simulink model "power_3phseriescomp"  (R2022a)
settings: Solver=FixedStepDiscrete  StartTime=0.0  StopTime=0.2  FixedStep=Ts  RelTol=1e-4  EnableMultiTasking=on
PreLoadFcn:
  | Ts=50e-6;
InitFcn:
  | Ts=50e-6;
undefined symbols (not defined in the file): D1, Delta, DiscIntNeverNeededParam
libraries: spsSeriesRLCBranchLib x6, spsBreakerLib x6, spsCurrentMeasurementLib x6, spsSurgeArresterLib x6, spsParallelRLCBranchLib x6, spsVoltageMeasurementLib x6, spsThreePhaseSeriesRLCLoadLib x4, spsLoadFlowBusLib x4, spsThreePhaseVIMeasurementLib x3, spsThreePhaseBreakerLib x2, spsDistributedParametersLineLib x2, spsThreePhaseSourceLib x1
(part 1 of 2)
settings Model: ExtModeTrigMode=oneshot  ExtModeArmWhenConnect=off  Creator=The MathWorks, Inc.  LastModifiedBy=thoma
settings SolverCC: AlgebraicLoopSolver=TrustRegion
settings DataIOCC: SaveFormat=Array  ReturnWorkspaceOutputs=off  SignalLoggingName=sigsOut
settings OptimizationCC: BlockReduction=off  BooleanDataType=off  ExpressionDepthLimit=2147483647  InitFltsAndDblsToZero=on  EfficientMapNaN2IntZero=off  LifeSpan=inf
settings DebuggingCC: UnderspecifiedInitializationDetection=Classic  MergeDetectMultiDrivingBlocksExec=none  CheckExecutionContextPreStartOutputMsg=on  SignalResolutionControl=TryResolveAllWithWarning  MultiTaskDSMMsg=warning  MultiTaskCondExecSysMsg=none  FcnCallInpInsideContextMsg=warning  UnconnectedLineMsg=warning  StateNameClashWarn=warning  SFUnexpectedBacktrackingDiag=warning  SFNoUnconditionalDefaultTransitionDiag=warning  SFExecutionAtInitializationDiag=none  SFMachineParentedDataDiag=warning  ArithmeticOperatorsInVariantConditions=warning
settings HardwareCC: ProdBitPerPointer=32  ProdBitPerSizeT=32  ProdBitPerPtrDiffT=32  ProdLargestAtomicFloat=None  ProdIntDivRoundTo=Undefined  ProdEndianess=Unspecified  ProdWordSize=32  ProdHWDeviceType=Specified  TargetUnknown=on
settings ModelReferenceCC: PropagateSignalLabelsOutOfModel=off
settings SFSimCC: SimUseLocalCustomCode=off  CustomCodeUndefinedFunction=UseInterfaceOnly
settings RTWCC: RTWUseLocalCustomCode=off  DLArmComputeVersion=19.05
settings CodeAppCC: StateflowObjectComments=on
settings GRTTargetCC: TargetLangStandard=C89/C90 (ANSI)  CombineOutputUpdateFcns=off  GRTInterface=on
settings ConfigComp: CovMetricSettings=dw  CovSaveCumulativeToWorkspaceVar=on  CovSaveSingleToWorkspaceVar=on  CovExternalEMLEnable=off  CovSFcnEnable=off
settings SimscapeCC: SimscapeNormalizeSystem=off

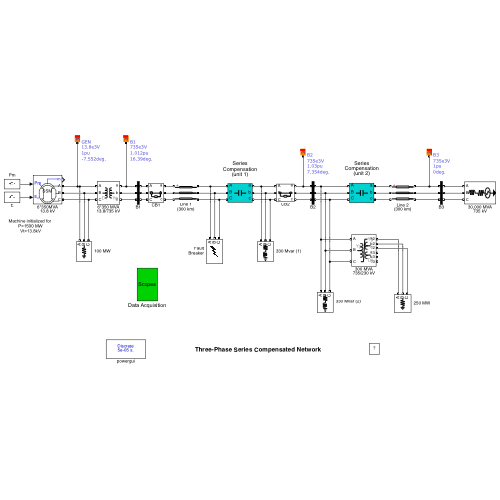
[thumbnail: Simulink's stored preview of the top-level diagram]
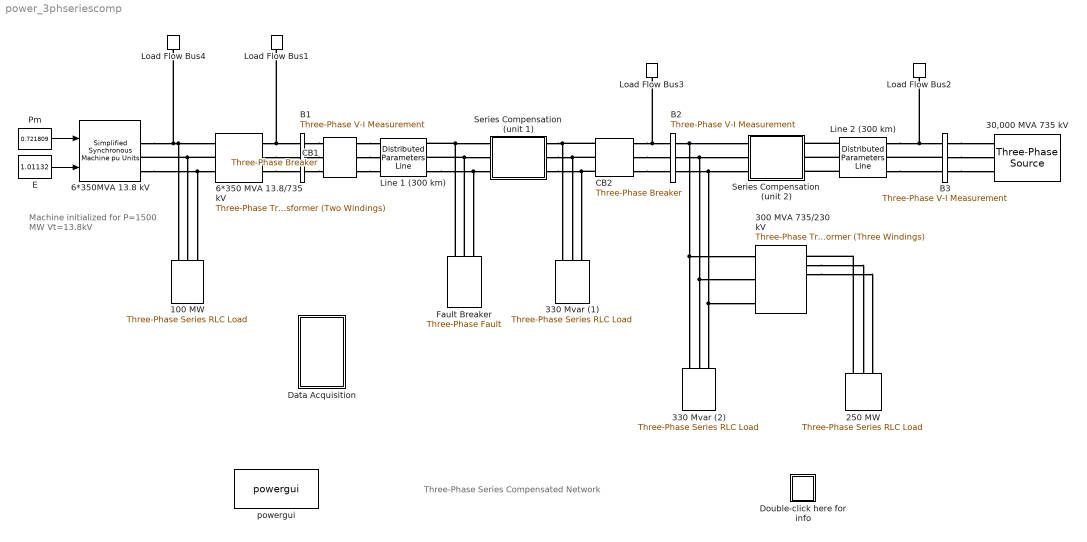
== system power_3phseriescomp ==
  note: Machine initialized for
      |  P=1500 MW
      |  Vt=13.8kV
  note: Three-Phase Series Compensated Network
  100 MW : spsThreePhaseSeriesRLCLoadLib/Three-Phase Series RLC Load  LConnTagsString=A|B|C  Configuration=Y (grounded)  NominalVoltage=13.8e3  Vabc=[1e3 1e3 1e3]  Vabcp=[1e3 1e3 1e3]  NominalFrequency=60  UnbalancedPower=off  ActivePower=100000000  InductivePower=0  CapacitivePower=0  Pabc=[10e3 9e3 11e3]  QLabc=[100 90 110]  QCabc=[100 90 110]  Pabcp=[10e3 9e3 11e3]  QLabcp=[100 90 110]  QCabcp=[100 90 110]  Measurements=None  LoadType=constant Z
  250 MW : spsThreePhaseSeriesRLCLoadLib/Three-Phase Series RLC Load  LConnTagsString=A|B|C  Configuration=Y (grounded)  NominalVoltage=230e3  Vabc=[1e3 1e3 1e3]  Vabcp=[1e3 1e3 1e3]  NominalFrequency=60  UnbalancedPower=off  ActivePower=250000000  InductivePower=0  CapacitivePower=0  Pabc=[10e3 9e3 11e3]  QLabc=[100 90 110]  QCabc=[100 90 110]  Pabcp=[10e3 9e3 11e3]  QLabcp=[100 90 110]  QCabcp=[100 90 110]  Measurements=None  LoadType=constant Z
  30,000 MVA 735 kV : spsThreePhaseSourceLib/Three-Phase Source  InternalConnection=Yg  VoltagePhases=off  Voltage=(735000)*0.98865  PhaseAngle=-2.0892  Voltage_phases=[25e3 25e3 25e3]/sqrt(3)  PhaseAngles_phases=[0 -120 +120]  Frequency=60  NonIdealSource=on  SpecifyImpedance=on  Resistance=735^2/30000/10  Inductance=735^2/30000/377  ShortCircuitLevel=30000e6  BaseVoltage=735e3  XRratio=10  BusType=swing  Pref=0  Qref=0  Prefabc=[10e3, 10e3, 10e3]  Qrefabc=[0, 0, 0]  Qmin=-Inf  Qmax=Inf
  300 MVA 735/230 kV : spsThreePhaseTransformerThreeWindingsLib/Three-Phase Transformer (Three Windings)  Winding1Connection=Yg  Winding2Connection=Yg  Winding3Connection=Delta (D1)  CoreType=Three single-phase transformers  SetSaturation=on  Hysteresis=off  DataFile='hysteresis'  SetInitialFlux=off  Measurements=None  UNITS=pu  NominalPower=[ 300e6 , 60 ]  Winding1=[ 735e3 , 0.002 , 0.15 ]  Winding2=[ 230e3 , 0.002 , 0 ]  Winding3=[ 25e3 , 0.05 , 0.20 ]  Rm=500  Lm=1000  L0=0.5  Saturation="[  0,0  ;  0.0012,1.2  ;  1.0,1.45 ]"  InitialFluxes=[-1.02015948080927 0.506449133666726 0.513710347142541]  BreakLoop=on  DiscreteSolver=Trapezoidal iterative  DataType=off  TransfoNumber=0
      settings: AttributesFormatString=\n  SourceProductBaseCode=PS
  330 Mvar (1) : spsThreePhaseSeriesRLCLoadLib/Three-Phase Series RLC Load  LConnTagsString=A|B|C  Configuration=Y (grounded)  NominalVoltage=735e3  Vabc=[1e3 1e3 1e3]  Vabcp=[1e3 1e3 1e3]  NominalFrequency=60  UnbalancedPower=off  ActivePower=1320000  InductivePower=330e6  CapacitivePower=0  Pabc=[10e3 9e3 11e3]  QLabc=[100 90 110]  QCabc=[100 90 110]  Pabcp=[10e3 9e3 11e3]  QLabcp=[100 90 110]  QCabcp=[100 90 110]  Measurements=None  LoadType=constant Z
  "330 Mvar (2) " : spsThreePhaseSeriesRLCLoadLib/Three-Phase Series RLC Load  LConnTagsString=A|B|C  Configuration=Y (grounded)  NominalVoltage=735e3  Vabc=[1e3 1e3 1e3]  Vabcp=[1e3 1e3 1e3]  NominalFrequency=60  UnbalancedPower=off  ActivePower=1320000  InductivePower=330e6  CapacitivePower=0  Pabc=[10e3 9e3 11e3]  QLabc=[100 90 110]  QCabc=[100 90 110]  Pabcp=[10e3 9e3 11e3]  QLabcp=[100 90 110]  QCabcp=[100 90 110]  Measurements=None  LoadType=constant Z
  6*350 MVA 13.8/735 kV : spsThreePhaseTransformerTwoWindingsLib/Three-Phase Transformer (Two Windings)  Winding1Connection=Delta (D1)  Winding2Connection=Yg  CoreType=Three single-phase transformers  SetSaturation=off  Hysteresis=off  DataFile='hysteresis'  SetInitialFlux=off  Measurements=None  UNITS=pu  NominalPower=[ 6*350e6 , 60 ]  Winding1=[ 13.8e3 , 0.002 , 0.08 ]  Winding2=[ 735e3 , 0.002 , 0.08 ]  Rm=500  Lm=500  L0=0.5  Saturation=[ 0,0 ; 0.0024,1.2 ; 1.0,1.52 ]  InitialFluxes=[ 0.8 , -0.8 , 0.7 ]  BreakLoop=off  DiscreteSolver=Trapezoidal iterative  DataType=off  TransfoNumber=0
  6*350MVA 13.8 kV : spsSimplifiedSynchronousMachinepuUnitsLib/Simplified Synchronous Machine pu Units  ConnectionType=3-wire Y  MechanicalLoad=Mechanical power Pm  MeasurementBus=off  NominalParameters="[ 6*350e6 13.8e3  60 ]"  Mechanical=[ inf,0,2 ]  InternalRL="[ 0.22/15  0.22 ]"  InitialConditions=[0 1.43122 0.716215 0.716215 0.716215 -3.34575 -123.346 116.654 ]  IterativeDiscreteModel=Trapezoidal non iterative  TsBlock=-1  TsPowergui=0  LoadFlowParameters=[1,0,0,0,0]  Units=0  BusType=PV  Pref=1500000000  Qref=0  Qmin=-Inf  Qmax=Inf  PLF=0  QLF=0
      settings: AttributesFormatString=\n  SourceProductBaseCode=PS
  B1 : spsThreePhaseVIMeasurementLib/Three-Phase V-I Measurement  VoltageMeasurement=phase-to-ground  SetLabelV=on  LabelV=Vabc_B1  Vpu=on  VpuLL=off  CurrentMeasurement=yes  SetLabelI=on  LabelI=Iabc_B1  Ipu=on  Pbase=100e6  Vbase=735e3  OutputType=Complex  PhasorSimulation=off  PSBequivalent=0
  B2 : spsThreePhaseVIMeasurementLib/Three-Phase V-I Measurement  VoltageMeasurement=phase-to-ground  SetLabelV=on  LabelV=Vabc_B2  Vpu=on  VpuLL=off  CurrentMeasurement=yes  SetLabelI=on  LabelI=Iabc_B2  Ipu=on  Pbase=100e6  Vbase=735e3  OutputType=Complex  PhasorSimulation=off  PSBequivalent=0
  B3 : spsThreePhaseVIMeasurementLib/Three-Phase V-I Measurement  VoltageMeasurement=no  SetLabelV=on  LabelV=Vabc_B3  Vpu=on  VpuLL=off  CurrentMeasurement=no  SetLabelI=on  LabelI=Iabc_B3  Ipu=on  Pbase=100e6  Vbase=735e3  OutputType=Complex  PhasorSimulation=off  PSBequivalent=0
  CB1 : spsThreePhaseBreakerLib/Three-Phase Breaker  InitialState=closed  SwitchA=on  SwitchB=on  SwitchC=on  SwitchTimes="[5/60  ]"  External=off  BreakerResistance=0.001  SnubberResistance=1e5  SnubberCapacitance=inf  Measurements=None
      settings: AttributesFormatString=\n
  CB2 : spsThreePhaseBreakerLib/Three-Phase Breaker  InitialState=closed  SwitchA=on  SwitchB=on  SwitchC=on  SwitchTimes="[5/60  ]"  External=off  BreakerResistance=0.001  SnubberResistance=1e5  SnubberCapacitance=inf  Measurements=None
      settings: AttributesFormatString=\n
  Data Acquisition : Subsystem  mask(Data Acquisition){}
      mask Display: disp('Scopes')
  Double-click here for info : Subsystem
      settings: OpenFcn=showdemo(bdroot(gcb))
      mask Display: disp('?')
  E : Constant  Value=1.01132
  Fault Breaker : spsThreePhaseFaultLib/Three-Phase Fault  InitialStates=0  FaultA=on  FaultB=off  FaultC=off  GroundFault=on  SwitchTimes=[ 1/60 6/60]  External=off  SwitchStatus=NaN  FaultResistance=0.001  GroundResistance=1  SnubberResistance=inf  SnubberCapacitance=inf  Measurements=Fault currents
  Line 1 (300 km) : spsDistributedParametersLineLib/Distributed Parameters Line  Phases=3  Length=300  Frequency=60  Resistance=[0.01273 0.3864]  Inductance="[0.9337e-3  4.1264e-3]"  Capacitance=[12.74e-9 7.751e-9]  x1=[-0.0017 -9.8128912515287e-08 0 0;-0.00165 -9.90072730950498e-08 0 0;-0.0016 -9.98504568621167e-08 0 0;-0.00155 -1.0065816423731e-07 0 0;-0.0015 -1.01430108246046e-07 0 0;-0.00145 -1.02166014620294e-07 0 0;-0.0014 -1.02865621896022e-07 0 0;-0.00135 -1.03528681506097e-07 0 0;-0.0013 -1.04154957868598e-07 0 0;-0.00125 -1.04744228470514e-07 0 0;-0.0012 -1.05296283946806e-07 0 0;-0.00115 -1.05810928154793e-07 0 0;-0.0011 -1.06287978243837e-07 0 0;-0.00105 -1.06727264720314e-07 298982.565692147 -680729.342896261;-0.001 -1.07128631507831e-07 311760.155284911 -674973.083751637;-0.00095 -1.07491936002678e-07 324426.977978985 -668977.009884319;-0.0009 -1.07817049124499e-07 336978.53331258 -662743.251670802;-0.00085 -1.0810385536215e-07 349410.361777853 -656274.023935697;-0.0008 -1.0835225281474e-07 361718.046405344 -649571.625164814;-0.00075 -1.08562153227837e-07 373897.214333311 -642638.436688521;-0.0007 -1.08733482024824e-07 385943.538361381 -635476.921835672;-0.00065 -1.08866178333394e-07 397852.738487986 -628089.625058393;-0.0006 -1.08960195007182e-07 409620.58343103 -620479.171028054;-0.00055 -1.0901549864251e-07 421242.892131238 -612648.263702733;-0.0005 -1.09032069590261e-07 432715.535237669 -604599.685366516;-0.00045 -1.09009901962856e-07 444034.436574856 -596336.29564096;-0.0004 -1.08949003636347e-07 455195.57459105 -587861.03046909;-0.00035 -1.08849396247619e-07 466194.98378706 -579176.901072263;-0.0003 -1.08711115186704e-07 477028.756125173 -570286.992880304;-0.00025 -1.08534209584204e-07 487693.042417663 -561194.464435264;-0.0002 -1.08318742293837e-07 498184.05369439 -551902.546269203;-0.00015 -1.08064789870105e-07 508498.062549001 -542414.539756403;-0.0001 -1.07772442541096e-07 518631.404463263 -532733.815940397;-5e-05 -1.07441804176423e-07 528580.479109043 -522863.814336263]  x2=[-0.0017 -2.91100446537141e-08 0 0;-0.00165 -2.9400539946736e-08 0 0;-0.0016 -2.9680589367909e-08 0 0;-0.00155 -2.99500934170071e-08 0 0;-0.0015 -3.02089563405251e-08 0 0;-0.00145 -3.04570861656989e-08 0 0;-0.0014 -3.06943947331829e-08 0 0;-0.00135 -3.09207977283733e-08 0 0;-0.0013 -3.11362147113638e-08 0 0;-0.00125 -3.13405691455261e-08 0 0;-0.0012 -3.15337884247028e-08 0 0;-0.00115 -3.17158038990041e-08 0 0;-0.0011 -3.18865508991986e-08 0 0;-0.00105 -3.20459687596902e-08 112715.556110755 -734159.055210882;-0.001 -3.21940008400721e-08 126533.290927804 -731904.127817147;-0.00095 -3.23305945452511e-08 140306.06906909 -729389.158371847;-0.0009 -3.24557013441342e-08 154028.997132119 -726615.04043165;-0.00085 -3.25692767868712e-08 167697.199425895 -723582.759627452;-0.0008 -3.26712805206484e-08 181305.819703225 -720293.393314181;-0.00075 -3.27616763040248e-08 194850.022886123 -716748.110188029;-0.0007 -3.28404320198089e-08 208324.996783692 -712948.169871207;-0.00065 -3.29075196864699e-08 221725.953801867 -708894.922464418;-0.0006 -3.29629154680794e-08 235048.13264443 -704589.808067163;-0.00055 -3.300659968278e-08 248286.800004675 -700034.356266089;-0.0005 -3.3038556809778e-08 261437.252247124 -695230.185591531;-0.00045 -3.30587754948585e-08 274494.817078715 -690179.002942452;-0.0004 -3.30672485544189e-08 287454.855208837 -684882.602979997;-0.00035 -3.30639729780216e-08 300312.761997653 -679342.867489852;-0.0003 -3.30489499294632e-08 313063.969092107 -673561.764713659;-0.00025 -3.30221847463613e-08 325703.946049033 -667541.348649707;-0.0002 -3.29836869382581e-08 338228.201944805 -661283.758323157;-0.00015 -3.29334701832414e-08 350632.28697094 -654791.217026056;-0.0001 -3.28715523230852e-08 362911.794015091 -648066.031527411;-5e-05 -3.27979553569104e-08 375062.360226877 -641110.591253607]  x3=[-0.0017 -1.31188382446923e-10 0 0;-0.00165 -1.30142334975837e-10 0 0;-0.0016 -1.29050048552822e-10 0 0;-0.00155 -1.27911911262044e-10 0 0;-0.0015 -1.26728327478262e-10 0 0;-0.00145 -1.25499717723158e-10 0 0;-0.0014 -1.24226518515929e-10 0 0;-0.00135 -1.22909182218191e-10 0 0;-0.0013 -1.21548176873258e-10 0 0;-0.00125 -1.20143986039847e-10 0 0;-0.0012 -1.18697108620276e-10 0 0;-0.00115 -1.17208058683202e-10 0 0;-0.0011 -1.15677365280979e-10 0 0;-0.00105 -1.14105572261682e-10 21.8468552412687 -927.93157658473;-0.001 -1.12493238075888e-10 39.3329301227214 -927.355137167546;-0.00095 -1.10840935578256e-10 56.8050302013898 -926.449212885838;-0.0009 -1.09149251823995e-10 74.2569477233117 -925.214125610188;-0.00085 -1.07418787860287e-10 91.6824821052906 -923.650314161226;-0.0008 -1.05650158512741e-10 109.075442137934 -921.758334153712;-0.00075 -1.0384399216694e-10 126.429648185362 -919.538857799134;-0.0007 -1.02000930545188e-10 143.7389343808 -916.992673666873;-0.00065 -1.00121628478502e-10 160.997150817281 -914.120686404027;-0.0006 -9.82067536739595e-11 178.198165732685 -910.923916413995;-0.00055 -9.62569864774593e-11 195.335867688315 -907.403499493933;-0.0005 -9.42730196320027e-11 212.40416774027 -903.560686431209;-0.00045 -9.2255558031563e-11 229.397001602814 -899.396842559008;-0.0004 -9.02053184706404e-11 246.30833180299 -894.913447271229;-0.00035 -8.81230293895884e-11 263.132149825703 -890.112093496871;-0.0003 -8.60094306158025e-11 279.862478248517 -884.994487134068;-0.00025 -8.38652731008629e-11 296.493372865408 -879.562446443991;-0.0002 -8.16913186537249e-11 313.018924798708 -873.817901404833;-0.00015 -7.94883396700521e-11 329.433262598503 -867.762893026093;-0.0001 -7.72571188577877e-11 345.730554328733 -861.399572623416;-5e-05 -7.4998448959062e-11 361.905009639246 -854.730201054242]  x4=[-0.0017 4.1359961743659e-12 0 0;-0.00165 6.47865374332128e-13 0 0;-0.0016 -2.84049560918428e-12 0 0;-0.00155 -6.32784737813608e-12 0 0;-0.0015 -9.81295089304523e-12 0 0;-0.00145 -1.32945679132276e-11 0 0;-0.0014 -1.67714614367341e-11 0 0;-0.00135 -2.02423961398514e-11 0 0;-0.0013 -2.37061388160067e-11 0 0;-0.00125 -2.71614588139203e-11 0 0;-0.0012 -3.06071284748498e-11 0 0;-0.00115 -3.40419235687717e-11 0 0;-0.0011 -3.74646237293442e-11 0 0;-0.00105 -4.08740128874979e-11 457.510949143639 -4541.09394571609;-0.001 -4.42688797034991e-11 543.022422494241 -4531.66378032673;-0.00095 -4.76480179973331e-11 628.340962563795 -4520.62353637426;-0.0009 -5.10102271772544e-11 713.436256081271 -4507.97713640481;-0.00085 -5.43543126663507e-11 798.278069094071 -4493.72907362406;-0.0008 -5.76790863269713e-11 882.836257710018 -4477.88441030087;-0.00075 -6.09833668828656e-11 967.080778807329 -4460.44877596867;-0.0007 -6.42659803388859e-11 1050.9817007088 -4441.42836542533;-0.00065 -6.75257603981019e-11 1134.50921381638 -4420.82993653213;-0.0006 -7.07615488761803e-11 1217.63364120239 -4398.66080781279;-0.00055 -7.39721961128824e-11 1300.32544915359 -4374.92885585317;-0.0005 -7.71565613805331e-11 1382.55525766436 -4349.64251250282;-0.00045 -8.03135132893152e-11 1464.29385087528 -4322.8107618791;-0.0004 -8.3441930189248e-11 1545.5121874534 -4294.44313717526;-0.00035 -8.65407005687031e-11 1626.18141091044 -4264.54971727328;-0.0003 -8.96087234493199e-11 1706.27285985545 -4233.14112316292;-0.00025 -9.26449087771777e-11 1785.75807817797 -4200.22851416809;-0.0002 -9.56481778100866e-11 1864.60882515841 -4165.82358398206;-0.00015 -9.86174635008596e-11 1942.79708550183 -4129.93855651271;-0.0001 -1.0155171087643e-10 2020.29507929163 -4092.58618153941;-5e-05 -1.04449877412676e-10 2097.07527185962 -4053.77973018315]  x5=0.00169662470098723  V1=ones(3,3)  V2=ones(3,3)  I1=ones(3,3)  I2=ones(3,3)  nHarmo=1  Measurements=None  Decoupling=off  VsMag0=0  VrMag0=0  VsAngle0=0  VrAngle0=0  IsMag0=0  IrMag0=0  IsAngle0=0  IrAngle0=0
      settings: AttributesFormatString=\n  SourceProductBaseCode=PS
  Line 2 (300 km) : spsDistributedParametersLineLib/Distributed Parameters Line  Phases=3  Length=300  Frequency=60  Resistance=[0.01273 0.3864]  Inductance="[0.9337e-3  4.1264e-3]"  Capacitance=[12.74e-9 7.751e-9]  x1=[-0.0017 -3.83784847275404e-08 0 0;-0.00165 -3.867993227856e-08 0 0;-0.0016 -3.896763703382e-08 0 0;-0.00155 -3.92414967731909e-08 0 0;-0.0015 -3.95014141956114e-08 0 0;-0.00145 -3.97472969536587e-08 0 0;-0.0014 -3.99790576863599e-08 0 0;-0.00135 -4.01966140502302e-08 0 0;-0.0013 -4.03998887485293e-08 0 0;-0.00125 -4.05888095587249e-08 0 0;-0.0012 -4.07633093581526e-08 0 0;-0.00115 -4.09233261478648e-08 0 0;-0.0011 -4.10688030746578e-08 0 0;-0.00105 -4.11996884512724e-08 246177.226114312 -694466.011958518;-0.001 -4.13159357747574e-08 259223.108712892 -689702.607076715;-0.00095 -4.14175037429923e-08 272176.890575268 -684694.154142718;-0.0009 -4.15043562693617e-08 285033.969284425 -679442.432636007;-0.00085 -4.15764624955765e-08 297789.776781518 -673949.308468225;-0.0008 -4.16337968026378e-08 310439.780988881 -668216.733320234;-0.00075 -4.16763388199394e-08 322979.487420255 -662246.743948687;-0.0007 -4.17040734325051e-08 335404.440777654 -656041.461462381;-0.00065 -4.17169907863591e-08 347710.226534312 -649603.090568636;-0.0006 -4.17150862920271e-08 359892.472503146 -642933.918789974;-0.00055 -4.16983606261668e-08 371946.850390169 -636036.315651371;-0.0005 -4.16668197313277e-08 383869.077332318 -628912.73183838;-0.00045 -4.16204748138395e-08 395654.917419129 -621565.698326408;-0.0004 -4.15593423398308e-08 407300.183197738 -613997.82548148;-0.00035 -4.14834440293784e-08 418800.737160666 -606211.802132781;-0.0003 -4.13928068487907e-08 430152.493215849 -598210.394617334;-0.00025 -4.12874630010264e-08 441351.418138414 -589996.445797128;-0.0002 -4.1167449914253e-08 452393.533003661 -581572.874049068;-0.00015 -4.10328102285487e-08 463274.914600758 -572942.672228087;-0.0001 -4.08835917807527e-08 473991.696826635 -564108.906603797;-5e-05 -4.07198475874691e-08 484540.072059597 -555074.715771062]  x2=[-0.0017 -1.55480927351862e-09 0 0;-0.00165 -1.55928375561788e-09 0 0;-0.0016 -1.56320423162349e-09 0 0;-0.00155 -1.56656930860897e-09 0 0;-0.0015 -1.56937779097852e-09 0 0;-0.00145 -1.5716286808917e-09 0 0;-0.0014 -1.57332117861807e-09 0 0;-0.00135 -1.57445468282122e-09 0 0;-0.0013 -1.57502879077252e-09 0 0;-0.00125 -1.57504329849414e-09 0 0;-0.0012 -1.57449820083156e-09 0 0;-0.00115 -1.57339369145539e-09 0 0;-0.0011 -1.57173016279254e-09 0 0;-0.00105 -1.56950820588683e-09 93647.54895747 -729009.85235218;-0.001 -1.56672861018896e-09 107371.613342243 -727115.238496599;-0.00095 -1.56339236327606e-09 121057.529104058 -724962.284059026;-0.0009 -1.55950065050077e-09 134700.433702212 -722551.753973919;-0.00085 -1.5550548545701e-09 148295.479877664 -719884.504691142;-0.0008 -1.55005655505417e-09 161837.837375241 -716961.483871662;-0.00075 -1.54450752782502e-09 175322.694659809 -713783.73005086;-0.0007 -1.53840974442558e-09 188745.260625785 -710352.372269536;-0.00065 -1.53176537136926e-09 202100.766299392 -706668.629672772;-0.0006 -1.52457676937018e-09 215384.46653306 -702733.81107677;-0.00055 -1.5168464925044e-09 228591.641691348 -698549.314503843;-0.0005 -1.50857728730247e-09 241717.599327809 -694116.626685698;-0.00045 -1.49977209177364e-09 254757.675852195 -689437.32253521;-0.0004 -1.49043403436193e-09 267707.23818741 -684513.064586862;-0.00035 -1.4805664328347e-09 280561.685415616 -679345.602406056;-0.0003 -1.47017279310377e-09 293316.450412922 -673936.7719675;-0.00025 -1.45925680797986e-09 305967.001472057 -668288.495002893;-0.0002 -1.44782235586049e-09 318508.843912467 -662402.778318146;-0.00015 -1.43587349935206e-09 330937.521677253 -656281.713080372;-0.0001 -1.42341448382639e-09 343248.618916384 -649927.474074903;-5e-05 -1.41044973591238e-09 355437.761555633 -643342.318932601]  x3=[-0.0017 -5.57932988104945e-11 0 0;-0.00165 -5.49197230916592e-11 0 0;-0.0016 -5.40266346567161e-11 0 0;-0.00155 -5.31143508157337e-11 0 0;-0.0015 -5.21831956988167e-11 0 0;-0.00145 -5.12335001409443e-11 0 0;-0.0014 -5.02656015644263e-11 0 0;-0.00135 -4.9279843859018e-11 0 0;-0.0013 -4.82765772597383e-11 0 0;-0.00125 -4.72561582224329e-11 0 0;-0.0012 -4.62189492971269e-11 0 0;-0.00115 -4.51653189992126e-11 0 0;-0.0011 -4.40956416785178e-11 0 0;-0.00105 -4.30102973863013e-11 12.2377893957938 -1258.52081063277;-0.001 -4.1909671740222e-11 35.9566534775546 -1258.06675540884;-0.00095 -4.07941557873313e-11 59.6627423315466 -1257.16571505713;-0.0009 -3.96641458651355e-11 83.3476332972795 -1255.81800971302;-0.00085 -3.85200434607793e-11 107.002911245771 -1254.02411820977;-0.0008 -3.73622550683993e-11 130.620171569405 -1251.78467790851;-0.00075 -3.61911920446983e-11 154.191023168043 -1249.10048447171;-0.0007 -3.50072704627924e-11 177.707091430348 -1245.97249158052;-0.00065 -3.38109109643823e-11 201.160021209241 -1242.40181059591;-0.0006 -3.26025386103012e-11 224.541479790446 -1238.38971016384;-0.00055 -3.13825827294927e-11 247.843159853062 -1233.93761576449;-0.0005 -3.01514767664723e-11 271.056782421117 -1229.0471092058;-0.00045 -2.89096581273266e-11 294.174099805046 -1223.71992806146;-0.0004 -2.7657568024305e-11 317.186898532059 -1217.95796505356;-0.00035 -2.63956513190591e-11 340.087002264347 -1211.76326738014;-0.0003 -2.51243563645856e-11 362.866274704095 -1205.13803598776;-0.00025 -2.38441348459284e-11 385.516622484271 -1198.08462478961;-0.0002 -2.2555441619697e-11 408.029998044161 -1190.60553982909;-0.00015 -2.12587345524585e-11 430.398402488629 -1182.70343838948;-0.0001 -1.99544743580596e-11 452.613888430085 -1174.38112804979;-5e-05 -1.86431244339368e-11 474.668562812157 -1165.64156568726]  x4=[-0.0017 1.37497058522874e-11 0 0;-0.00165 1.21949628669792e-11 0 0;-0.0016 1.06358870694321e-11 0 0;-0.00155 9.07303239185332e-12 0 0;-0.0015 7.506954109068e-12 0 0;-0.00145 5.93820864123296e-12 0 0;-0.0014 4.36735335614317e-12 0 0;-0.00135 2.79494637120162e-12 0 0;-0.0013 1.22154635512285e-12 0 0;-0.00125 -3.52287670559359e-13 0 0;-0.0012 -1.92599653010968e-12 0 0;-0.00115 -3.49902109226372e-12 0 0;-0.0011 -5.07080246888466e-12 0 0;-0.00105 -6.64078221353364e-12 198.236296947625 -4189.81019371945;-0.001 -8.20840251988303e-12 277.17266159117 -4185.32933734589;-0.00095 -9.77310641990236e-12 356.010548107841 -4179.3614533877;-0.0009 -1.13343379817465e-11 434.721945771956 -4171.90866220565;-0.00085 -1.28915425072755e-11 513.278888798718 -4162.97361174096;-0.0008 -1.44441667291363e-11 591.653466280328 -4152.5594765745;-0.00075 -1.59916590073359e-11 669.817832102597 -4140.66995679892;-0.0007 -1.75334695252363e-11 747.744214838536 -4127.30927670398;-0.00065 -1.9069050484902e-11 825.404927615415 -4112.48218327569;-0.0006 -2.05978563017301e-11 902.772377951775 -4096.19394450975;-0.00055 -2.21193437982932e-11 979.819077560906 -4078.45034753985;-0.0005 -2.36329723973287e-11 1056.51765211731 -4059.25769658148;-0.00045 -2.51382043138025e-11 1132.84085098264 -4038.62281069215;-0.0004 -2.66345047459823e-11 1208.76155688778 -4016.55302134856;-0.00035 -2.81213420654491e-11 1284.25279556741 -3993.05616984178;-0.0003 -2.95981880059831e-11 1359.2877453439 -3968.14060449126;-0.00025 -3.10645178512539e-11 1433.83974665688 -3941.81517767874;-0.0002 -3.25198106212495e-11 1507.88231153527 -3914.08924270301;-0.00015 -3.39635492573783e-11 1581.38913300833 -3884.97265045674;-0.0001 -3.53952208061774e-11 1654.3340944524 -3854.47574592652;-5e-05 -3.68143166015625e-11 1726.69127887002 -3822.60936451731]  x5=0.00169662470098723  V1=ones(3,3)  V2=ones(3,3)  I1=ones(3,3)  I2=ones(3,3)  nHarmo=1  Measurements=None  Decoupling=off  VsMag0=0  VrMag0=0  VsAngle0=0  VrAngle0=0  IsMag0=0  IrMag0=0  IsAngle0=0  IrAngle0=0
      settings: AttributesFormatString=\n  SourceProductBaseCode=PS
  Load Flow Bus1 : spsLoadFlowBusLib/Load Flow Bus  LConnTagsString=a  Phases=single  Connectors=on one side  ID=B1  Vbase=735e3  Vref=1  Vangle=0  VLF=1.012  VLFb=1  VLFc=1  angleLF=16.39  angleLFb=0  angleLFc=0
      settings: AttributesFormatString=%<ID>\n%<Vbase>V\n%<VLF>pu\n%<angleLF>deg.  SourceProductBaseCode=PS
  Load Flow Bus2 : spsLoadFlowBusLib/Load Flow Bus  LConnTagsString=a  Phases=single  Connectors=on one side  ID=B3  Vbase=735e3  Vref=1  Vangle=0  VLF=1  VLFb=1  VLFc=1  angleLF=0  angleLFb=0  angleLFc=0
      settings: AttributesFormatString=%<ID>\n%<Vbase>V\n%<VLF>pu\n%<angleLF>deg.  SourceProductBaseCode=PS
  Load Flow Bus3 : spsLoadFlowBusLib/Load Flow Bus  LConnTagsString=a  Phases=single  Connectors=on one side  ID=B2  Vbase=735e3  Vref=1  Vangle=0  VLF=1.03  VLFb=1  VLFc=1  angleLF=7.354  angleLFb=0  angleLFc=0
      settings: AttributesFormatString=%<ID>\n%<Vbase>V\n%<VLF>pu\n%<angleLF>deg.  SourceProductBaseCode=PS
  Load Flow Bus4 : spsLoadFlowBusLib/Load Flow Bus  LConnTagsString=a  Phases=single  Connectors=on one side  ID=GEN  Vbase=13.8e3  Vref=1  Vangle=0  VLF=1  VLFb=1  VLFc=1  angleLF=-7.552  angleLFb=0  angleLFc=0
      settings: AttributesFormatString=%<ID>\n%<Vbase>V\n%<VLF>pu\n%<angleLF>deg.  SourceProductBaseCode=PS
  Pm : Constant  Value=0.721809
  "Series Compensation (unit 1) " : Subsystem
      mask Display: plot(0,0,100,100,[25 45],[50 50], [45 45],[35 65],[55 55],[35 65], [55 75],[50 50])
  "Series Compensation (unit 2) " : Subsystem
      mask Display: plot(0,0,100,100,[25 45],[50 50], [45 45],[35 65],[55 55],[35 65], [55 75],[50 50])
  powergui : spspowerguiLib/powergui  Priority=2  SimulationMode=Discrete  SampleTime=Ts  frequency=60  Iterations=50  frequencyindice=60  Pbase=100e6  ErrMax=0.0001  UnitsV=kV  UnitsW=MW  buscounter=0  FunctionMessages=off  echomessages=off  EnableUseOfTLC=off  CurrentSourceSwitches=off  DisableSnubberDevices=off  DisableRonSwitches=off  DisableVfSwitches=off  DisplayEquations=off  AutomaticDiscreteSolvers=off  SolverType=Tustin/Backward Euler (TBE)  Interpol=off  ExternalGateDelay=off  methode=off  Ts=0  x0status=blocks  SPID=off  SwTol=0  HookPort=off  NonlinearTolerance=1e-4  nMaxIteration=100  ContinueOnMaxIteration=off  RestoreLinks=warning  ResistiveCurrentMeasurement=off  Frange=0:0.5:500  Ylog=off  Xlog=off  ShowGrid=off  save=on  variable=Zmes  structure=0  ZoomFFT=on  StartTime=0.0  cycles=1  DisplayStyle=off  fundamental=60  FreqAxis=off  MaxFrequency=1000  frequencyindicesteady=1  RmsSteady=1  display=off
  wires:
  Pm/1 -> 6*350MVA 13.8 kV/1
  E/1 -> 6*350MVA 13.8 kV/2
  connections:
  6*350 MVA 13.8/735 kV/LConn2 -- 6*350MVA 13.8 kV/RConn2 -- 100 MW/LConn2
  6*350MVA 13.8 kV/RConn1 -- 6*350 MVA 13.8/735 kV/LConn1 -- 100 MW/LConn1 -- Load Flow Bus4/LConn1
  6*350MVA 13.8 kV/RConn3 -- 6*350 MVA 13.8/735 kV/LConn3 -- 100 MW/LConn3
  6*350 MVA 13.8/735 kV/RConn2 -- B1/LConn2
  6*350 MVA 13.8/735 kV/RConn1 -- B1/LConn1 -- Load Flow Bus1/LConn1
  6*350 MVA 13.8/735 kV/RConn3 -- B1/LConn3
  B1/RConn2 -- CB1/LConn2
  B1/RConn1 -- CB1/LConn1
  B1/RConn3 -- CB1/LConn3
  CB1/RConn2 -- Line 1 (300 km)/LConn2
  CB1/RConn1 -- Line 1 (300 km)/LConn1
  CB1/RConn3 -- Line 1 (300 km)/LConn3
  Fault Breaker/LConn2 -- Line 1 (300 km)/RConn2 -- "Series Compensation (unit 1) "/LConn2
  Fault Breaker/LConn1 -- Line 1 (300 km)/RConn1 -- "Series Compensation (unit 1) "/LConn1
  Line 1 (300 km)/RConn3 -- Fault Breaker/LConn3 -- "Series Compensation (unit 1) "/LConn3
  CB2/RConn2 -- B2/LConn2
  CB2/RConn1 -- B2/LConn1 -- Load Flow Bus3/LConn1
  CB2/RConn3 -- B2/LConn3
  CB2/LConn2 -- 330 Mvar (1)/LConn2 -- "Series Compensation (unit 1) "/RConn2
  CB2/LConn3 -- 330 Mvar (1)/LConn3 -- "Series Compensation (unit 1) "/RConn3
  CB2/LConn1 -- 330 Mvar (1)/LConn1 -- "Series Compensation (unit 1) "/RConn1
  B2/RConn2 -- "330 Mvar (2) "/LConn2 -- 300 MVA 735/230 kV/LConn2 -- "Series Compensation (unit 2) "/LConn2
  B2/RConn3 -- "330 Mvar (2) "/LConn3 -- 300 MVA 735/230 kV/LConn3 -- "Series Compensation (unit 2) "/LConn3
  B2/RConn1 -- "330 Mvar (2) "/LConn1 -- 300 MVA 735/230 kV/LConn1 -- "Series Compensation (unit 2) "/LConn1
  300 MVA 735/230 kV/RConn2 -- 250 MW/LConn2
  250 MW/LConn1 -- 300 MVA 735/230 kV/RConn1
  300 MVA 735/230 kV/RConn3 -- 250 MW/LConn3
  Line 2 (300 km)/RConn1 -- B3/LConn1 -- Load Flow Bus2/LConn1
  B3/LConn2 -- Line 2 (300 km)/RConn2
  Line 2 (300 km)/RConn3 -- B3/LConn3
  B3/RConn3 -- 30,000 MVA 735 kV/RConn3
  B3/RConn2 -- 30,000 MVA 735 kV/RConn2
  B3/RConn1 -- 30,000 MVA 735 kV/RConn1
  Line 2 (300 km)/LConn2 -- "Series Compensation (unit 2) "/RConn2
  Line 2 (300 km)/LConn1 -- "Series Compensation (unit 2) "/RConn1
  Line 2 (300 km)/LConn3 -- "Series Compensation (unit 2) "/RConn3

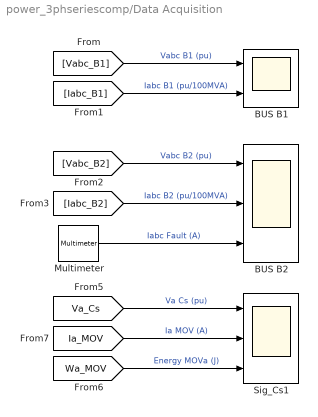
== system power_3phseriescomp/Data Acquisition ==
  BUS B1 : Scope  NumInputPorts=2
  BUS B2 : Scope  NumInputPorts=3
  Multimeter : spsMultimeterLib/Multimeter  Tag=PoWeRsYsTeMmEaSuReMeNt  L=3  sel=1  yselected={'Ib: Fault Breaker/Fault A'};  Gain=1  OutputType=Magnitude  PlotAtSimulationStop=off  PhasorSimulation=off
      settings: AttributesFormatString=\n
  Sig_Cs1 : Scope  NumInputPorts=3
  wires:
  [Vabc_B1] -> BUS B1/1  "Vabc B1 (pu)"
  [Iabc_B1] -> BUS B1/2  "Iabc B1 (pu/100MVA)"
  [Vabc_B2] -> BUS B2/1  "Vabc B2 (pu)"
  [Iabc_B2] -> BUS B2/2  "Iabc B2 (pu/100MVA)"
  [Va_Cs] -> Sig_Cs1/1  "Va Cs (pu)"
  [Ia_MOV] -> Sig_Cs1/2  "Ia MOV (A)"
  [Wa_MOV] -> Sig_Cs1/3  "Energy MOVa (J)"
  Multimeter/1 -> BUS B2/3  "Iabc Fault (A)"

== system power_3phseriescomp/Double-click here for info ==

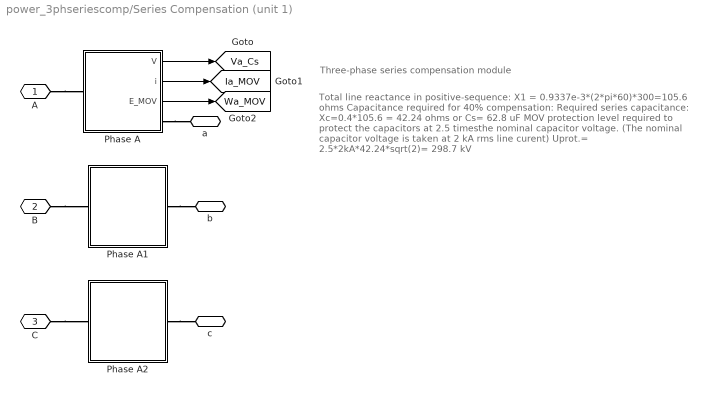
== system power_3phseriescomp/Series Compensation (unit 1)  ==
  note: Three-phase series compensation module
  note: Total line reactance in positive-sequence:
      |  X1 = 0.9337e-3*(2*pi*60)*300=105.6 ohms
      |
      | Capacitance required for 40% compensation:
      |
      | Required series capacitance:
      | Xc=0.4*105.6 = 42.24 ohms
      | or Cs= 62.8 uF
      |
      | MOV protection level required to protect the capacitors
      | at 2.5 timesthe nominal capacitor voltage.
      | (The nominal capacitor voltage is taken at 2 kA  rms line curent)
      |
      | Uprot.= 2.5*2kA*42.24*sqrt(2)= 298.7 kV
  Phase A : Subsystem
  Phase A1 : Subsystem
  Phase A2 : Subsystem
  A : PMIOPort  Side=Left
  B : PMIOPort  Port=2  Side=Left
  C : PMIOPort  Port=3  Side=Left
  a : PMIOPort  Port=4  Side=Right
  b : PMIOPort  Port=5  Side=Right
  c : PMIOPort  Port=6  Side=Right
  tag scope: Ia_MOV=global, Va_Cs=global, Wa_MOV=global
  wires:
  Phase A/2(i) -> [Ia_MOV]
  Phase A/1(V) -> [Va_Cs]
  Phase A/3(E_MOV) -> [Wa_MOV]
  connections:
  A/RConn1 -- Phase A/LConn1
  B/RConn1 -- Phase A1/LConn1
  C/RConn1 -- Phase A2/LConn1
  Phase A/RConn1 -- a/RConn1
  Phase A1/RConn1 -- b/RConn1
  Phase A2/RConn1 -- c/RConn1

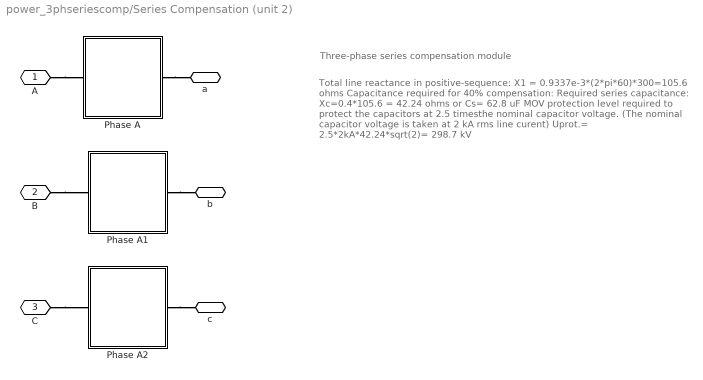
== system power_3phseriescomp/Series Compensation (unit 2)  ==
  note: Total line reactance in positive-sequence:
      |  X1 = 0.9337e-3*(2*pi*60)*300=105.6 ohms
      |
      | Capacitance required for 40% compensation:
      |
      | Required series capacitance:
      | Xc=0.4*105.6 = 42.24 ohms
      | or Cs= 62.8 uF
      |
      | MOV protection level required to protect the capacitors
      | at 2.5 timesthe nominal capacitor voltage.
      | (The nominal capacitor voltage is taken at 2 kA  rms line curent)
      |
      | Uprot.= 2.5*2kA*42.24*sqrt(2)= 298.7 kV
  note: Three-phase series compensation module
  Phase A : Subsystem
  Phase A1 : Subsystem
  Phase A2 : Subsystem
  A : PMIOPort  Side=Left
  B : PMIOPort  Port=2  Side=Left
  C : PMIOPort  Port=3  Side=Left
  a : PMIOPort  Port=4  Side=Right
  b : PMIOPort  Port=5  Side=Right
  c : PMIOPort  Port=6  Side=Right
  connections:
  Phase A2/RConn1 -- c/RConn1
  Phase A1/RConn1 -- b/RConn1
  Phase A/RConn1 -- a/RConn1
  C/RConn1 -- Phase A2/LConn1
  B/RConn1 -- Phase A1/LConn1
  A/RConn1 -- Phase A/LConn1

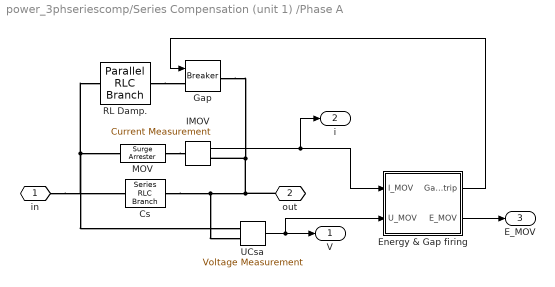
== system power_3phseriescomp/Series Compensation (unit 1) /Phase A ==
  Cs : spsSeriesRLCBranchLib/Series RLC Branch  LConnTagsString=__new0  RConnTagsString=__new0  BranchType=C  Resistance=1.0  Inductance=1.0  SetiL0=off  InitialCurrent=0  Capacitance=62.8e-6  Setx0=off  InitialVoltage=0  Measurements=None
  Energy & Gap firing : Subsystem
  Gap : spsBreakerLib/Breaker  InitialState=0  SwitchingTimes="[ 4/60  5/60 ]"  External=on  BreakerResistance=0.001  SnubberResistance=inf  SnubberCapacitance=0  Measurements=None  MoreParameters=off  NoBreakLoop=off
      settings: AttributesFormatString=\n  SourceProductBaseCode=PS
  IMOV : spsCurrentMeasurementLib/Current Measurement  Tag=PoWeRsYsTeMmEaSuReMeNt  PhasorSimulation=off  OutputType=Magnitude  PSBequivalent=0
      settings: AttributesFormatString=\n
  MOV : spsSurgeArresterLib/Surge Arrester  ProtectionVoltage=298.7e+03  Columns=60  ReferenceCurrent=500  Segment1=[.955 50]  Segment2=[1.0 25]  Segment3=[.9915 16.5]  Measurements=None  BreakLoop=on  UseDiscreteRobustSolver=on
      settings: AttributesFormatString=\n  SourceProductBaseCode=PS
  RL Damp. : spsParallelRLCBranchLib/Parallel RLC Branch  LConnTagsString=a  RConnTagsString=__new0  BranchType=RL  Resistance=7.5  Inductance=1.7e-3  SetiL0=off  InitialCurrent=0  Capacitance=1.0  Setx0=off  InitialVoltage=0  Measurements=None
  UCsa : spsVoltageMeasurementLib/Voltage Measurement  Tag=PoWeRsYsTeMmEaSuReMeNt  PhasorSimulation=off  OutputType=Magnitude  PSBequivalent=0
  in : PMIOPort  Side=Left
  "out " : PMIOPort  Port=2  Side=Right
  V : Outport  VectorParamsAs1DForOutWhenUnconnected=off
  i : Outport  Port=2  VectorParamsAs1DForOutWhenUnconnected=off
  E_MOV : Outport  Port=3  VectorParamsAs1DForOutWhenUnconnected=off
  wires:
  Energy & Gap firing/2(E_MOV) -> E_MOV/1
  IMOV/1 -> Energy & Gap firing/1(I_MOV), i/1
  UCsa/1 -> Energy & Gap firing/2(U_MOV), V/1
  Energy & Gap firing/1(Gap_trip) -> Gap/1
  connections:
  MOV/RConn1 -- IMOV/LConn1
  Cs/LConn1 -- UCsa/LConn1 -- in/RConn1 -- RL Damp./LConn1 -- MOV/LConn1
  RL Damp./RConn1 -- Gap/LConn1
  Cs/RConn1 -- "out "/RConn1 -- IMOV/RConn1 -- Gap/RConn1 -- UCsa/LConn2

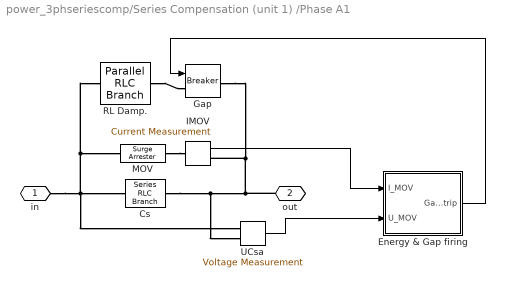
== system power_3phseriescomp/Series Compensation (unit 1) /Phase A1 ==
  Cs : spsSeriesRLCBranchLib/Series RLC Branch  LConnTagsString=__new0  RConnTagsString=__new0  BranchType=C  Resistance=1.0  Inductance=1.0  SetiL0=off  InitialCurrent=0  Capacitance=62.8e-6  Setx0=off  InitialVoltage=0  Measurements=None
  Energy & Gap firing : Subsystem
  Gap : spsBreakerLib/Breaker  InitialState=0  SwitchingTimes="[ 4/60  5/60 ]"  External=on  BreakerResistance=0.001  SnubberResistance=inf  SnubberCapacitance=0  Measurements=None  MoreParameters=off  NoBreakLoop=off
      settings: AttributesFormatString=\n  SourceProductBaseCode=PS
  IMOV : spsCurrentMeasurementLib/Current Measurement  Tag=PoWeRsYsTeMmEaSuReMeNt  PhasorSimulation=off  OutputType=Magnitude  PSBequivalent=0
      settings: AttributesFormatString=\n
  MOV : spsSurgeArresterLib/Surge Arrester  ProtectionVoltage=298.7e+03  Columns=60  ReferenceCurrent=500  Segment1=[.955 50]  Segment2=[1.0 25]  Segment3=[.9915 16.5]  Measurements=None  BreakLoop=on  UseDiscreteRobustSolver=on
      settings: AttributesFormatString=\n  SourceProductBaseCode=PS
  RL Damp. : spsParallelRLCBranchLib/Parallel RLC Branch  LConnTagsString=a  RConnTagsString=__new0  BranchType=RL  Resistance=7.5  Inductance=1.7e-3  SetiL0=off  InitialCurrent=0  Capacitance=1.0  Setx0=off  InitialVoltage=0  Measurements=None
  UCsa : spsVoltageMeasurementLib/Voltage Measurement  Tag=PoWeRsYsTeMmEaSuReMeNt  PhasorSimulation=off  OutputType=Magnitude  PSBequivalent=0
  in : PMIOPort  Side=Left
  "out " : PMIOPort  Port=2  Side=Right
  wires:
  Energy & Gap firing/1(Gap_trip) -> Gap/1
  UCsa/1 -> Energy & Gap firing/2(U_MOV)
  IMOV/1 -> Energy & Gap firing/1(I_MOV)
  connections:
  "out "/RConn1 -- UCsa/LConn2 -- Cs/RConn1 -- Gap/RConn1 -- IMOV/RConn1
  RL Damp./RConn1 -- Gap/LConn1
  in/RConn1 -- UCsa/LConn1 -- Cs/LConn1 -- MOV/LConn1 -- RL Damp./LConn1
  MOV/RConn1 -- IMOV/LConn1

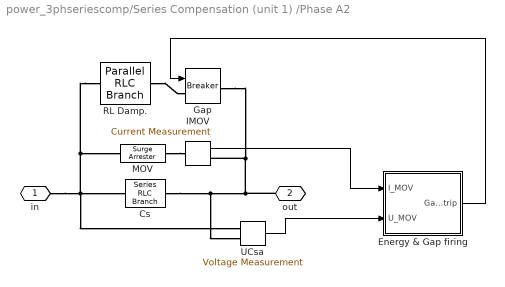
== system power_3phseriescomp/Series Compensation (unit 1) /Phase A2 ==
  Cs : spsSeriesRLCBranchLib/Series RLC Branch  LConnTagsString=__new0  RConnTagsString=__new0  BranchType=C  Resistance=1.0  Inductance=1.0  SetiL0=off  InitialCurrent=0  Capacitance=62.8e-6  Setx0=off  InitialVoltage=0  Measurements=None
  Energy & Gap firing : Subsystem
  Gap : spsBreakerLib/Breaker  InitialState=0  SwitchingTimes="[ 4/60  5/60 ]"  External=on  BreakerResistance=0.001  SnubberResistance=inf  SnubberCapacitance=0  Measurements=None  MoreParameters=off  NoBreakLoop=off
      settings: AttributesFormatString=\n  SourceProductBaseCode=PS
  IMOV : spsCurrentMeasurementLib/Current Measurement  Tag=PoWeRsYsTeMmEaSuReMeNt  PhasorSimulation=off  OutputType=Magnitude  PSBequivalent=0
      settings: AttributesFormatString=\n
  MOV : spsSurgeArresterLib/Surge Arrester  ProtectionVoltage=298.7e+03  Columns=60  ReferenceCurrent=500  Segment1=[.955 50]  Segment2=[1.0 25]  Segment3=[.9915 16.5]  Measurements=None  BreakLoop=on  UseDiscreteRobustSolver=on
      settings: AttributesFormatString=\n  SourceProductBaseCode=PS
  RL Damp. : spsParallelRLCBranchLib/Parallel RLC Branch  LConnTagsString=a  RConnTagsString=__new0  BranchType=RL  Resistance=7.5  Inductance=1.7e-3  SetiL0=off  InitialCurrent=0  Capacitance=1.0  Setx0=off  InitialVoltage=0  Measurements=None
  UCsa : spsVoltageMeasurementLib/Voltage Measurement  Tag=PoWeRsYsTeMmEaSuReMeNt  PhasorSimulation=off  OutputType=Magnitude  PSBequivalent=0
  in : PMIOPort  Side=Left
  "out " : PMIOPort  Port=2  Side=Right
  wires:
  IMOV/1 -> Energy & Gap firing/1(I_MOV)
  UCsa/1 -> Energy & Gap firing/2(U_MOV)
  Energy & Gap firing/1(Gap_trip) -> Gap/1
  connections:
  MOV/RConn1 -- IMOV/LConn1
  RL Damp./LConn1 -- MOV/LConn1 -- Cs/LConn1 -- UCsa/LConn1 -- in/RConn1
  RL Damp./RConn1 -- Gap/LConn1
  IMOV/RConn1 -- Gap/RConn1 -- Cs/RConn1 -- UCsa/LConn2 -- "out "/RConn1

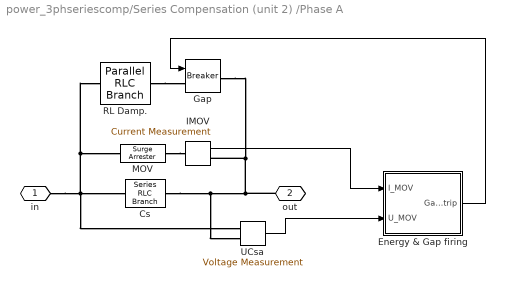
== system power_3phseriescomp/Series Compensation (unit 2) /Phase A ==
  Cs : spsSeriesRLCBranchLib/Series RLC Branch  LConnTagsString=__new0  RConnTagsString=__new0  BranchType=C  Resistance=1.0  Inductance=1.0  SetiL0=off  InitialCurrent=0  Capacitance=62.8e-6  Setx0=off  InitialVoltage=0  Measurements=None
  Energy & Gap firing : Subsystem
  Gap : spsBreakerLib/Breaker  InitialState=0  SwitchingTimes="[ 4/60  5/60 ]"  External=on  BreakerResistance=0.001  SnubberResistance=inf  SnubberCapacitance=0  Measurements=None  MoreParameters=off  NoBreakLoop=off
      settings: AttributesFormatString=\n  SourceProductBaseCode=PS
  IMOV : spsCurrentMeasurementLib/Current Measurement  Tag=PoWeRsYsTeMmEaSuReMeNt  PhasorSimulation=off  OutputType=Magnitude  PSBequivalent=0
      settings: AttributesFormatString=\n
  MOV : spsSurgeArresterLib/Surge Arrester  ProtectionVoltage=298.7e+03  Columns=60  ReferenceCurrent=500  Segment1=[.955 50]  Segment2=[1.0 25]  Segment3=[.9915 16.5]  Measurements=None  BreakLoop=on  UseDiscreteRobustSolver=on
      settings: AttributesFormatString=\n  SourceProductBaseCode=PS
  RL Damp. : spsParallelRLCBranchLib/Parallel RLC Branch  LConnTagsString=a  RConnTagsString=__new0  BranchType=RL  Resistance=7.5  Inductance=1.7e-3  SetiL0=off  InitialCurrent=0  Capacitance=1.0  Setx0=off  InitialVoltage=0  Measurements=None
  UCsa : spsVoltageMeasurementLib/Voltage Measurement  Tag=PoWeRsYsTeMmEaSuReMeNt  PhasorSimulation=off  OutputType=Magnitude  PSBequivalent=0
  in : PMIOPort  Side=Left
  "out " : PMIOPort  Port=2  Side=Right
  wires:
  Energy & Gap firing/1(Gap_trip) -> Gap/1
  UCsa/1 -> Energy & Gap firing/2(U_MOV)
  IMOV/1 -> Energy & Gap firing/1(I_MOV)
  connections:
  "out "/RConn1 -- UCsa/LConn2 -- Cs/RConn1 -- Gap/RConn1 -- IMOV/RConn1
  RL Damp./RConn1 -- Gap/LConn1
  in/RConn1 -- UCsa/LConn1 -- Cs/LConn1 -- MOV/LConn1 -- RL Damp./LConn1
  MOV/RConn1 -- IMOV/LConn1

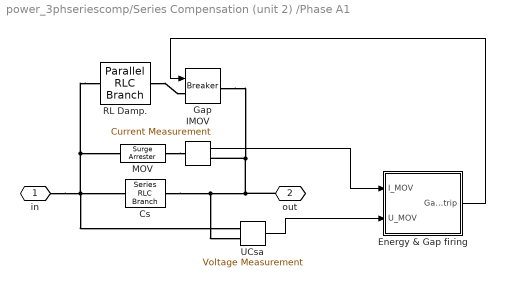
== system power_3phseriescomp/Series Compensation (unit 2) /Phase A1 ==
  Cs : spsSeriesRLCBranchLib/Series RLC Branch  LConnTagsString=__new0  RConnTagsString=__new0  BranchType=C  Resistance=1.0  Inductance=1.0  SetiL0=off  InitialCurrent=0  Capacitance=62.8e-6  Setx0=off  InitialVoltage=0  Measurements=None
  Energy & Gap firing : Subsystem
  Gap : spsBreakerLib/Breaker  InitialState=0  SwitchingTimes="[ 4/60  5/60 ]"  External=on  BreakerResistance=0.001  SnubberResistance=inf  SnubberCapacitance=0  Measurements=None  MoreParameters=off  NoBreakLoop=off
      settings: AttributesFormatString=\n  SourceProductBaseCode=PS
  IMOV : spsCurrentMeasurementLib/Current Measurement  Tag=PoWeRsYsTeMmEaSuReMeNt  PhasorSimulation=off  OutputType=Magnitude  PSBequivalent=0
      settings: AttributesFormatString=\n
  MOV : spsSurgeArresterLib/Surge Arrester  ProtectionVoltage=298.7e+03  Columns=60  ReferenceCurrent=500  Segment1=[.955 50]  Segment2=[1.0 25]  Segment3=[.9915 16.5]  Measurements=None  BreakLoop=on  UseDiscreteRobustSolver=on
      settings: AttributesFormatString=\n  SourceProductBaseCode=PS
  RL Damp. : spsParallelRLCBranchLib/Parallel RLC Branch  LConnTagsString=a  RConnTagsString=__new0  BranchType=RL  Resistance=7.5  Inductance=1.7e-3  SetiL0=off  InitialCurrent=0  Capacitance=1.0  Setx0=off  InitialVoltage=0  Measurements=None
  UCsa : spsVoltageMeasurementLib/Voltage Measurement  Tag=PoWeRsYsTeMmEaSuReMeNt  PhasorSimulation=off  OutputType=Magnitude  PSBequivalent=0
  in : PMIOPort  Side=Left
  "out " : PMIOPort  Port=2  Side=Right
  wires:
  IMOV/1 -> Energy & Gap firing/1(I_MOV)
  UCsa/1 -> Energy & Gap firing/2(U_MOV)
  Energy & Gap firing/1(Gap_trip) -> Gap/1
  connections:
  MOV/RConn1 -- IMOV/LConn1
  RL Damp./LConn1 -- MOV/LConn1 -- Cs/LConn1 -- UCsa/LConn1 -- in/RConn1
  RL Damp./RConn1 -- Gap/LConn1
  IMOV/RConn1 -- Gap/RConn1 -- Cs/RConn1 -- UCsa/LConn2 -- "out "/RConn1

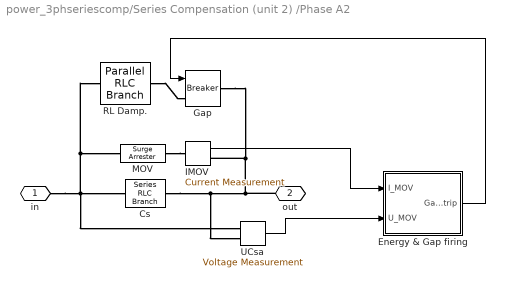
== system power_3phseriescomp/Series Compensation (unit 2) /Phase A2 ==
  Cs : spsSeriesRLCBranchLib/Series RLC Branch  LConnTagsString=__new0  RConnTagsString=__new0  BranchType=C  Resistance=1.0  Inductance=1.0  SetiL0=off  InitialCurrent=0  Capacitance=62.8e-6  Setx0=off  InitialVoltage=0  Measurements=None
  Energy & Gap firing : Subsystem
  Gap : spsBreakerLib/Breaker  InitialState=0  SwitchingTimes="[ 4/60  5/60 ]"  External=on  BreakerResistance=0.001  SnubberResistance=inf  SnubberCapacitance=0  Measurements=None  MoreParameters=off  NoBreakLoop=off
      settings: AttributesFormatString=\n  SourceProductBaseCode=PS
  IMOV : spsCurrentMeasurementLib/Current Measurement  Tag=PoWeRsYsTeMmEaSuReMeNt  PhasorSimulation=off  OutputType=Magnitude  PSBequivalent=0
      settings: AttributesFormatString=\n
  MOV : spsSurgeArresterLib/Surge Arrester  ProtectionVoltage=298.7e+03  Columns=60  ReferenceCurrent=500  Segment1=[.955 50]  Segment2=[1.0 25]  Segment3=[.9915 16.5]  Measurements=None  BreakLoop=on  UseDiscreteRobustSolver=on
      settings: AttributesFormatString=\n  SourceProductBaseCode=PS
  RL Damp. : spsParallelRLCBranchLib/Parallel RLC Branch  LConnTagsString=a  RConnTagsString=__new0  BranchType=RL  Resistance=7.5  Inductance=1.7e-3  SetiL0=off  InitialCurrent=0  Capacitance=1.0  Setx0=off  InitialVoltage=0  Measurements=None
  UCsa : spsVoltageMeasurementLib/Voltage Measurement  Tag=PoWeRsYsTeMmEaSuReMeNt  PhasorSimulation=off  OutputType=Magnitude  PSBequivalent=0
  in : PMIOPort  Side=Left
  "out " : PMIOPort  Port=2  Side=Right
  wires:
  Energy & Gap firing/1(Gap_trip) -> Gap/1
  UCsa/1 -> Energy & Gap firing/2(U_MOV)
  IMOV/1 -> Energy & Gap firing/1(I_MOV)
  connections:
  "out "/RConn1 -- UCsa/LConn2 -- Cs/RConn1 -- Gap/RConn1 -- IMOV/RConn1
  RL Damp./RConn1 -- Gap/LConn1
  in/RConn1 -- UCsa/LConn1 -- Cs/LConn1 -- MOV/LConn1 -- RL Damp./LConn1
  MOV/RConn1 -- IMOV/LConn1

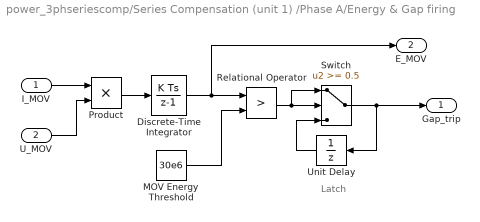
== system power_3phseriescomp/Series Compensation (unit 1) /Phase A/Energy & Gap firing ==
  note: Latch
  I_MOV : Inport
  U_MOV : Inport  Port=2
  Discrete-Time Integrator : DiscreteIntegrator  SampleTime=Ts  ICPrevOutput=DiscIntNeverNeededParam  ICPrevScaledInput=DiscIntNeverNeededParam
  MOV Energy Threshold : Constant  Value=30e6
  Product : Product  InputSameDT=on  SaturateOnIntegerOverflow=on  OutDataTypeStr=Inherit: Same as first input
  Relational Operator : RelationalOperator  Operator=>  ZeroCross=off
  Switch : Switch  Threshold=0.5  ZeroCross=off  SaturateOnIntegerOverflow=off
  Unit Delay : UnitDelay  SampleTime=Ts  HasFrameUpgradeWarning=on
  Gap_trip : Outport  VectorParamsAs1DForOutWhenUnconnected=off
  E_MOV : Outport  Port=2  InitialOutput=0  VectorParamsAs1DForOutWhenUnconnected=off
  wires:
  Switch/1 -> Unit Delay/1, Gap_trip/1
  U_MOV/1 -> Product/2
  MOV Energy Threshold/1 -> Relational Operator/2
  Product/1 -> Discrete-Time Integrator/1
  I_MOV/1 -> Product/1
  Discrete-Time Integrator/1 -> E_MOV/1, Relational Operator/1
  Relational Operator/1 -> Switch/1, Switch/2
  Unit Delay/1 -> Switch/3

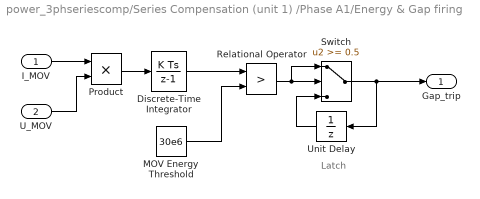
== system power_3phseriescomp/Series Compensation (unit 1) /Phase A1/Energy & Gap firing ==
  note: Latch
  I_MOV : Inport
  U_MOV : Inport  Port=2
  Discrete-Time Integrator : DiscreteIntegrator  SampleTime=Ts  ICPrevOutput=DiscIntNeverNeededParam  ICPrevScaledInput=DiscIntNeverNeededParam
  MOV Energy Threshold : Constant  Value=30e6
  Product : Product  InputSameDT=on  SaturateOnIntegerOverflow=on  OutDataTypeStr=Inherit: Same as first input
  Relational Operator : RelationalOperator  Operator=>  ZeroCross=off
  Switch : Switch  Threshold=0.5  ZeroCross=off  SaturateOnIntegerOverflow=off
  Unit Delay : UnitDelay  SampleTime=Ts  HasFrameUpgradeWarning=on
  Gap_trip : Outport  VectorParamsAs1DForOutWhenUnconnected=off
  wires:
  Unit Delay/1 -> Switch/3
  Relational Operator/1 -> Switch/2, Switch/1
  Discrete-Time Integrator/1 -> Relational Operator/1
  I_MOV/1 -> Product/1
  Product/1 -> Discrete-Time Integrator/1
  MOV Energy Threshold/1 -> Relational Operator/2
  U_MOV/1 -> Product/2
  Switch/1 -> Gap_trip/1, Unit Delay/1

== system power_3phseriescomp/Series Compensation (unit 1) /Phase A2/Energy & Gap firing ==
  note: Latch
  I_MOV : Inport
  U_MOV : Inport  Port=2
  Discrete-Time Integrator : DiscreteIntegrator  SampleTime=Ts  ICPrevOutput=DiscIntNeverNeededParam  ICPrevScaledInput=DiscIntNeverNeededParam
  MOV Energy Threshold : Constant  Value=30e6
  Product : Product  InputSameDT=on  SaturateOnIntegerOverflow=on  OutDataTypeStr=Inherit: Same as first input
  Relational Operator : RelationalOperator  Operator=>  ZeroCross=off
  Switch : Switch  Threshold=0.5  ZeroCross=off  SaturateOnIntegerOverflow=off
  Unit Delay : UnitDelay  SampleTime=Ts  HasFrameUpgradeWarning=on
  Gap_trip : Outport  VectorParamsAs1DForOutWhenUnconnected=off
  wires:
  Switch/1 -> Unit Delay/1, Gap_trip/1
  U_MOV/1 -> Product/2
  MOV Energy Threshold/1 -> Relational Operator/2
  Product/1 -> Discrete-Time Integrator/1
  I_MOV/1 -> Product/1
  Discrete-Time Integrator/1 -> Relational Operator/1
  Relational Operator/1 -> Switch/1, Switch/2
  Unit Delay/1 -> Switch/3

== system power_3phseriescomp/Series Compensation (unit 2) /Phase A/Energy & Gap firing ==
  note: Latch
  I_MOV : Inport
  U_MOV : Inport  Port=2
  Discrete-Time Integrator : DiscreteIntegrator  SampleTime=Ts  ICPrevOutput=DiscIntNeverNeededParam  ICPrevScaledInput=DiscIntNeverNeededParam
  MOV Energy Threshold : Constant  Value=30e6
  Product : Product  InputSameDT=on  SaturateOnIntegerOverflow=on  OutDataTypeStr=Inherit: Same as first input
  Relational Operator : RelationalOperator  Operator=>  ZeroCross=off
  Switch : Switch  Threshold=0.5  ZeroCross=off  SaturateOnIntegerOverflow=off
  Unit Delay : UnitDelay  SampleTime=Ts  HasFrameUpgradeWarning=on
  Gap_trip : Outport  VectorParamsAs1DForOutWhenUnconnected=off
  wires:
  Unit Delay/1 -> Switch/3
  Relational Operator/1 -> Switch/2, Switch/1
  Discrete-Time Integrator/1 -> Relational Operator/1
  I_MOV/1 -> Product/1
  Product/1 -> Discrete-Time Integrator/1
  MOV Energy Threshold/1 -> Relational Operator/2
  U_MOV/1 -> Product/2
  Switch/1 -> Gap_trip/1, Unit Delay/1

== system power_3phseriescomp/Series Compensation (unit 2) /Phase A1/Energy & Gap firing ==
  note: Latch
  I_MOV : Inport
  U_MOV : Inport  Port=2
  Discrete-Time Integrator : DiscreteIntegrator  SampleTime=Ts  ICPrevOutput=DiscIntNeverNeededParam  ICPrevScaledInput=DiscIntNeverNeededParam
  MOV Energy Threshold : Constant  Value=30e6
  Product : Product  InputSameDT=on  SaturateOnIntegerOverflow=on  OutDataTypeStr=Inherit: Same as first input
  Relational Operator : RelationalOperator  Operator=>  ZeroCross=off
  Switch : Switch  Threshold=0.5  ZeroCross=off  SaturateOnIntegerOverflow=off
  Unit Delay : UnitDelay  SampleTime=Ts  HasFrameUpgradeWarning=on
  Gap_trip : Outport  VectorParamsAs1DForOutWhenUnconnected=off
  wires:
  Switch/1 -> Unit Delay/1, Gap_trip/1
  U_MOV/1 -> Product/2
  MOV Energy Threshold/1 -> Relational Operator/2
  Product/1 -> Discrete-Time Integrator/1
  I_MOV/1 -> Product/1
  Discrete-Time Integrator/1 -> Relational Operator/1
  Relational Operator/1 -> Switch/1, Switch/2
  Unit Delay/1 -> Switch/3
